simulink model "manifold_blocks"  (R2018a)
settings: Solver=ode45  StartTime=0.0  StopTime=10.0  MaxStep=0.2  RelTol=1e-3  EnableMultiTasking=on
InitFcn:
  | load manifold_press_start.mat
settings Model: Creator=dlange  LastModifiedBy=bneiswan
settings DataIOCC: ExternalInput=[t, mdot_in, w]  LimitDataPoints=on  LoadExternalInput=on  SaveFormat=Array
settings OptimizationCC: ExpressionDepthLimit=2147483647  InitFltsAndDblsToZero=on  LifeSpan=inf
settings DebuggingCC: SaveWithParameterizedLinksMsg=none  UnderspecifiedInitializationDetection=Classic  MergeDetectMultiDrivingBlocksExec=none  SignalResolutionControl=TryResolveAllWithWarning  ParameterPrecisionLossMsg=none  FcnCallInpInsideContextMsg=warning  AllowSymbolicDim=off  StateNameClashWarn=warning  SFUnexpectedBacktrackingDiag=warning  SFNoUnconditionalDefaultTransitionDiag=warning  SFExecutionAtInitializationDiag=none
settings HardwareCC: ProdBitPerPointer=32  ProdBitPerSizeT=32  ProdBitPerPtrDiffT=32  ProdLargestAtomicFloat=None  ProdIntDivRoundTo=Undefined  ProdEndianess=Unspecified  ProdWordSize=32  ProdHWDeviceType=32-bit Generic
settings ModelReferenceCC: PropagateSignalLabelsOutOfModel=off
settings CodeAppCC: StateflowObjectComments=on
settings GRTTargetCC: TargetFcnLib=ansi_tfl_tmw.mat  TargetLangStandard=C89/C90 (ANSI)  GeneratePreprocessorConditionals=Disable all  CombineOutputUpdateFcns=off  GRTInterface=on
settings ConfigComp: CovMetricSettings=dw  CovHtmlReporting=on  CovSaveCumulativeToWorkspaceVar=on  CovSaveSingleToWorkspaceVar=on  CovExternalEMLEnable=off  CovSFcnEnable=off

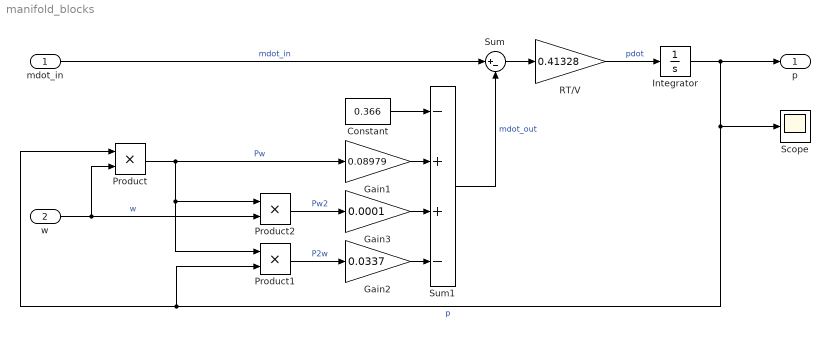
== system manifold_blocks ==
  mdot_in : Inport
  w : Inport  Port=2
  Constant : Constant  Value=0.366
  Gain1 : Gain  Gain=0.08979
  Gain2 : Gain  Gain=0.0337
  Gain3 : Gain  Gain=0.0001
  Integrator : Integrator  InitialCondition=0.543
      settings: AttributesFormatString=p0 = %<InitialCondition>
  Product : Product  RndMeth=Zero
  Product1 : Product  RndMeth=Zero
  Product2 : Product  RndMeth=Zero
  RT/V : Gain  Gain=0.41328
  Scope : Scope
  Sum : Sum  Inputs=|+-
  Sum1 : Sum  Inputs=-++-
  p : Outport
  wires:
  Integrator/1 -> p/1, Scope/1, Product/1, Product1/2  "p"
  RT/V/1 -> Integrator/1  "pdot"
  mdot_in/1 -> Sum/1  "mdot_in"
  Sum/1 -> RT/V/1
  Constant/1 -> Sum1/1
  Gain1/1 -> Sum1/2
  Product/1 -> Gain1/1, Product1/1, Product2/1  "Pw"
  Product1/1 -> Gain2/1  "P2w"
  Product2/1 -> Gain3/1  "Pw2"
  Sum1/1 -> Sum/2  "mdot_out"
  Gain3/1 -> Sum1/3
  Gain2/1 -> Sum1/4
  w/1 -> Product/2, Product2/2  "w"
